simulink model "ToWorkSpace"  (R2014a)
settings: Solver=ode45  StartTime=0.0  StopTime=2e-8  RelTol=1e-3
libraries: dspstat3 x1, simulink_extras x1
settings Model: Creator=Kushal  LastModifiedBy=Kushal
settings SolverCC: AutoInsertRateTranBlk=on  InsertRTBMode=Always

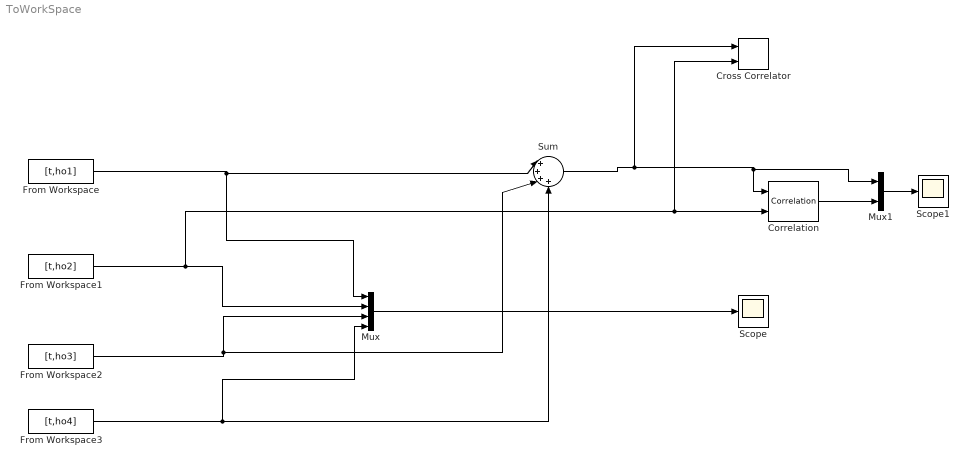
== system ToWorkSpace ==
  Correlation : dspstat3/Correlation  domain=Time  outputDataTypeStr=Inherit: Same as accumulator  outputLastDataTypeStr=Inherit: Same as accumulator  outputMin=[]  outputMax=[]  roundingMode=Floor  overflowMode=off
  Cross Correlator : simulink_extras/Additional Sinks/Cross Correlator  npts=6500  HowOften=6500  sampleT=20e-9
  From Workspace : FromWorkspace  VariableName=[t,ho1]  SampleTime=0
  From Workspace1 : FromWorkspace  VariableName=[t,ho2]  SampleTime=0
  From Workspace2 : FromWorkspace  VariableName=[t,ho3]  SampleTime=0
  From Workspace3 : FromWorkspace  VariableName=[t,ho4]  SampleTime=0
  Mux : Mux
  Mux1 : Mux  Inputs=2
  Scope : Scope
  Scope1 : Scope
  Sum : Sum  Inputs=|++++
  wires:
  From Workspace/1 -> Sum/1, Mux/1
  From Workspace1/1 -> Cross Correlator/2, Correlation/2, Mux/2
  From Workspace3/1 -> Sum/4, Mux/4
  Mux/1 -> Scope/1
  From Workspace2/1 -> Sum/3, Mux/3
  Sum/1 -> Cross Correlator/1, Mux1/1, Correlation/1
  Mux1/1 -> Scope1/1
  Correlation/1 -> Mux1/2
